simulink model "Projectile"  (R2022b)
settings: Solver=VariableStepAuto  StartTime=0.0  StopTime=2  RelTol=1e-3
settings Model: Creator=ASUS  LastModifiedBy=ASUS

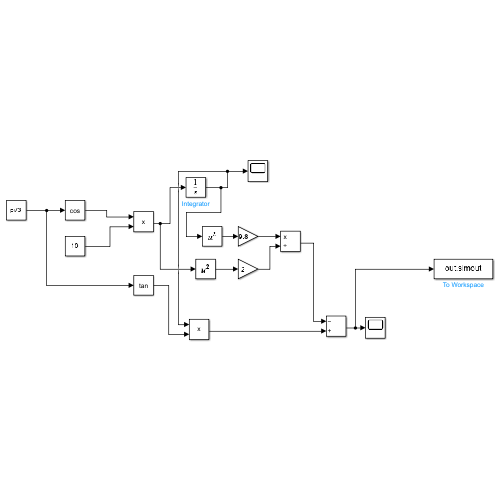
[thumbnail: Simulink's stored preview of the top-level diagram]
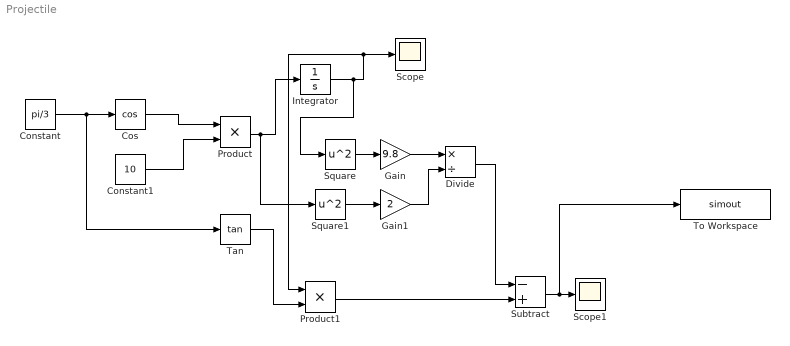
== system Projectile ==
  Constant : Constant  Value=pi/3
  Constant1 : Constant  Value=10
  Cos : Trigonometry  Operator=cos
  Divide : Product  Inputs=*/
  Gain : Gain  Gain=9.8
  Gain1 : Gain  Gain=2
  Integrator : Integrator
  Product : Product
  Product1 : Product
  Scope : Scope
  Scope1 : Scope
  Square : Math  Operator=square
  Square1 : Math  Operator=square
  Subtract : Sum  Inputs=-+
  Tan : Trigonometry  Operator=tan
  To Workspace : ToWorkspace  VariableName=simout  SaveFormat=Timeseries  SampleTime=-1
  wires:
  Constant/1 -> Tan/1, Cos/1
  Cos/1 -> Product/1
  Product/1 -> Square1/1, Integrator/1
  Constant1/1 -> Product/2
  Tan/1 -> Product1/2
  Product1/1 -> Subtract/2
  Square/1 -> Gain/1
  Gain/1 -> Divide/1
  Square1/1 -> Gain1/1
  Gain1/1 -> Divide/2
  Divide/1 -> Subtract/1
  Subtract/1 -> To Workspace/1, Scope1/1
  Integrator/1 -> Square/1, Product1/1, Scope/1
